simulink model "CalcRef_simulink"  (R2012b)
settings: Solver=ode45  StartTime=0.0  StopTime=15  RelTol=1e-3
values from neighbouring files (symbols this model uses):
  radio = 0.1    [matlab.mat]
  Ts = 0.06    [matlab.mat]
settings Model: Creator=Carlos  LastModifiedBy=Carlos

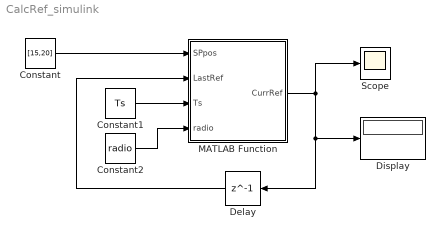
== system CalcRef_simulink ==
  Constant : Constant  Value=[15,20]
  Constant1 : Constant  Value=Ts
  Constant2 : Constant  Value=radio
  Delay : Delay  DelayLength=1  SampleTime=Ts
  Display : Display
  MATLAB Function : MATLAB Function  TreatAsAtomicUnit=on  RTWFcnName=CalcRef
  Scope : Scope
  wires:
  Constant/1 -> MATLAB Function/1(SPpos)
  Constant1/1 -> MATLAB Function/3(Ts)
  Constant2/1 -> MATLAB Function/4(radio)
  MATLAB Function/1(CurrRef) -> Scope/1, Delay/1, Display/1
  Delay/1 -> MATLAB Function/2(LastRef)

== matlab function CalcRef_simulink/MATLAB Function ==
  data: SPpos input; CurrRef output; LastRef input; Ts input; radio input
function CurrRef = CalcRef (SPpos, LastRef, Ts, radio)
%%bla bla bla

maxVx = 3;
maxVy = 1.85;

DistXY = SPpos -LastRef;

if (norm(DistXY)<(0.5*radio))
    CurrRef = LastRef + 0*DistXY;
else
        minTx=abs(DistXY(1))/maxVx;
        minTy=abs(DistXY(2))/maxVy;
        minT=max(minTx,minTy);
        %disp('minT')
        
        if minT<Ts
            CurrRef = SPpos;
        else
            CurrRef = LastRef+(Ts/minT)*DistXY;
        end
end
